simulink model "forcesmpc_onlinetuning"  (R2019b)
settings: Solver=ode3  StartTime=0.0  StopTime=10  RelTol=1e-3
values from neighbouring files (symbols this model uses):
  Ts = 1    [forcesmpc_cstr.m]    (also in forcesmpc_customqp.m = 0.2; forcesmpc_linearize.m = 0.1; forcesmpc_miso.m = 0.2; forcesmpc_motor.m = 0.1)
  v = -double(time>20)    [forcesmpc_preview.m]    (also in forcesmpc_run_onlinetuning.m = 0.5)
libraries: forceslib x1, cstblocks x1
settings Model: FPTRunName=Active  ExtModeTrigMode=oneshot  ExtModeArmWhenConnect=off  Creator=The MathWorks, Inc.  LastModifiedBy=j-hho
settings DataIOCC: SaveFormat=Array  ReturnWorkspaceOutputs=off  SignalLoggingName=sigsOut
settings OptimizationCC: BooleanDataType=off  ExpressionDepthLimit=2147483647  InitFltsAndDblsToZero=on  LifeSpan=inf
settings DebuggingCC: SaveWithParameterizedLinksMsg=none  UnderspecifiedInitializationDetection=Classic  MergeDetectMultiDrivingBlocksExec=none  SignalResolutionControl=TryResolveAllWithWarning  MultiTaskDSMMsg=warning  MultiTaskCondExecSysMsg=none  IntegerOverflowMsg=none  FcnCallInpInsideContextMsg=warning  StateNameClashWarn=warning  SFUnexpectedBacktrackingDiag=warning  SFNoUnconditionalDefaultTransitionDiag=warning  SFExecutionAtInitializationDiag=none  IntegerSaturationMsg=none  ArithmeticOperatorsInVariantConditions=warning
settings HardwareCC: ProdBitPerPointer=32  ProdBitPerSizeT=32  ProdBitPerPtrDiffT=32  ProdLargestAtomicInteger=Long  ProdWordSize=32  ProdHWDeviceType=ARM Compatible->ARM 10  TargetBitPerPointer=64  TargetBitPerSizeT=64  TargetBitPerPtrDiffT=64  TargetLongLongMode=on  TargetIntDivRoundTo=Zero  TargetEndianess=LittleEndian  TargetWordSize=64  TargetHWDeviceType=MATLAB Host  ProdEqTarget=off
settings ModelReferenceCC: PropagateSignalLabelsOutOfModel=off
settings SFSimCC: SimUseLocalCustomCode=off  CustomCodeUndefinedFunction=UseInterfaceOnly
settings RTWCC: GenCodeOnly=on  PackageGeneratedCodeAndArtifacts=on  RTWUseLocalCustomCode=off
settings CodeAppCC: StateflowObjectComments=on
settings GRTTargetCC: TargetFcnLib=ansi_tfl_tmw.mat  TargetLangStandard=C89/C90 (ANSI)  GeneratePreprocessorConditionals=Disable all  CombineOutputUpdateFcns=off  GRTInterface=on
settings ConfigComp: CovMetricSettings=dw  CovHtmlReporting=on  CovSaveCumulativeToWorkspaceVar=on  CovSaveSingleToWorkspaceVar=on  CovExternalEMLEnable=off  CovSFcnEnable=off

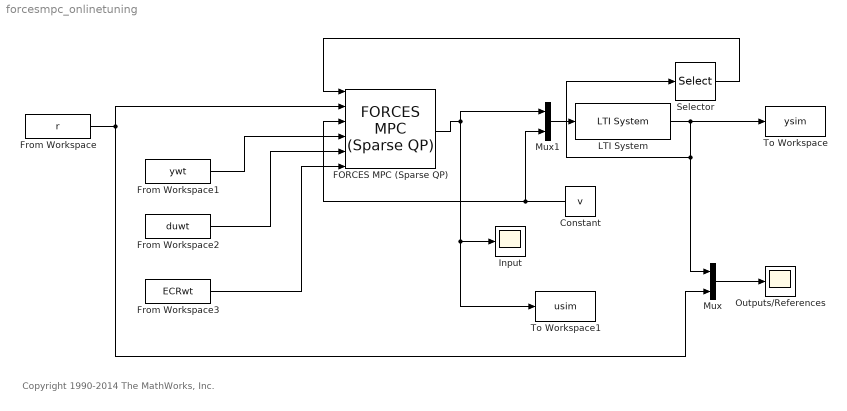
== system forcesmpc_onlinetuning ==
  note: Copyright 1990-2014 The MathWorks, Inc.
  Constant : Constant  Value=v
  FORCES MPC (Sparse QP) : forceslib/FORCES MPC (Sparse QP)  CoreData=coredata  StateData=statedata  md_inport=on  mv_inport=off  uref_inport=off  state_inport=off  ymin_inport=off  ymax_inport=off  umin_inport=off  umax_inport=off  dumin_inport=off  dumax_inport=off  ywt_inport=on  uwt_inport=off  duwt_inport=on  ecrwt_inport=on  return_cost=off  return_mvseq=off  return_qpstatus=off  return_xseq=off  return_state=off  return_yseq=off
  From Workspace : FromWorkspace  VariableName=r  SampleTime=Ts
  From Workspace1 : FromWorkspace  VariableName=ywt  SampleTime=Ts
  From Workspace2 : FromWorkspace  VariableName=duwt  SampleTime=Ts
  From Workspace3 : FromWorkspace  VariableName=ECRwt  SampleTime=Ts
  Input : Scope
  LTI System : cstblocks/LTI System  sys=plant  IC=[]
  Mux : Mux  Inputs=2
  Mux1 : Mux  Inputs=2
  Outputs/References : Scope
  Selector : Selector  InputPortWidth=4  IndexOptions=Index vector (dialog)  Indices=[1 2 3]  OutputSizes=1
  To Workspace : ToWorkspace  VariableName=ysim  SampleTime=-1
      settings: MaxDataPoints=Inf
  To Workspace1 : ToWorkspace  VariableName=usim  SampleTime=-1
      settings: MaxDataPoints=Inf
  wires:
  FORCES MPC (Sparse QP)/1 -> Input/1, To Workspace1/1, Mux1/1
  Mux/1 -> Outputs/References/1
  From Workspace/1 -> FORCES MPC (Sparse QP)/2, Mux/2
  LTI System/1 -> Selector/1, Mux/1, To Workspace/1
  Selector/1 -> FORCES MPC (Sparse QP)/1
  Mux1/1 -> LTI System/1
  Constant/1 -> FORCES MPC (Sparse QP)/3, Mux1/2
  From Workspace1/1 -> FORCES MPC (Sparse QP)/4
  From Workspace2/1 -> FORCES MPC (Sparse QP)/5
  From Workspace3/1 -> FORCES MPC (Sparse QP)/6
